simulink model "lqg_control"  (R2018a)
settings: Solver=ode45  StartTime=0.0  StopTime=10  RelTol=1e-3
settings Model: Creator=HARSH  LastModifiedBy=HARSH

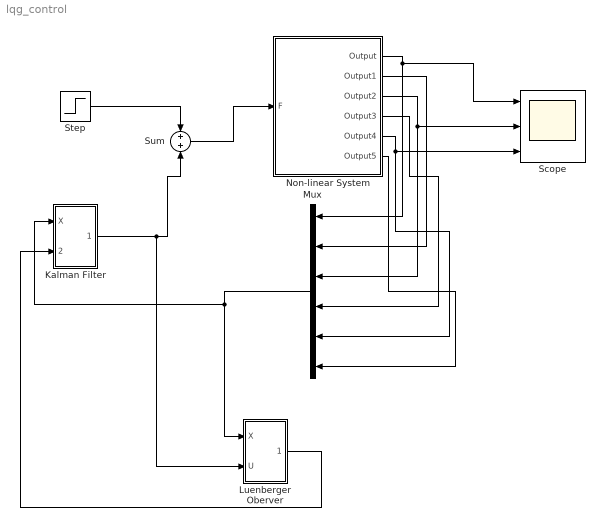
== system lqg_control ==
  "Kalman Filter " : Subsystem
  Luenberger Oberver : Subsystem
  Mux : Mux  Inputs=6
  Non-linear System : Subsystem
  Scope : Scope  NumInputPorts=3
  Step : Step  After=20  SampleTime=0
  Sum : Sum  Inputs=2
  wires:
  Non-linear System/1(Output) -> Scope/1, Mux/1
  Non-linear System/2(Output1) -> Mux/2
  Non-linear System/3(Output2) -> Scope/2, Mux/3
  Non-linear System/4(Output3) -> Mux/4
  Non-linear System/6(Output5) -> Mux/6
  Mux/1 -> "Kalman Filter "/1(X), Luenberger Oberver/1(X)
  Sum/1 -> Non-linear System/1(F)
  Step/1 -> Sum/1
  "Kalman Filter "/1(Out1) -> Luenberger Oberver/2(U), Sum/2
  Luenberger Oberver/1(X_hat) -> "Kalman Filter "/2(X_hat)
  Non-linear System/5(Output4) -> Scope/3, Mux/5

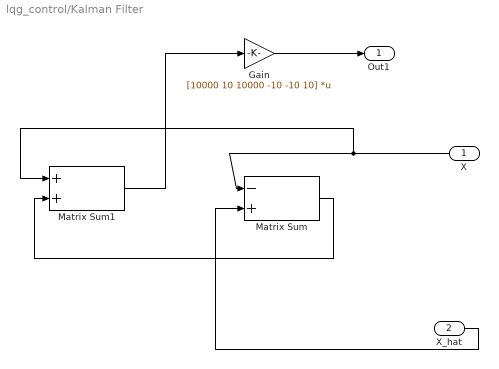
== system lqg_control/Kalman Filter  ==
  X : Inport
  X_hat : Inport  Port=2
  Gain : Gain  Gain=[10000 10 10000 -10 -10 10]  Multiplication=Matrix(K*u)
  Matrix Sum : Sum  Inputs=-+
  Matrix Sum1 : Sum  Inputs=2
  Out1 : Outport
  wires:
  X_hat/1 -> Matrix Sum/2
  Gain/1 -> Out1/1
  X/1 -> Matrix Sum1/1, Matrix Sum/1
  Matrix Sum/1 -> Matrix Sum1/2
  Matrix Sum1/1 -> Gain/1

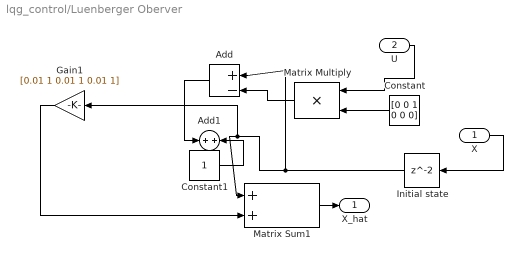
== system lqg_control/Luenberger Oberver ==
  X : Inport
  U : Inport  Port=2
  Add : Sum  Inputs=+|-
  Add1 : Sum
  Constant : Constant  Value=[0 0 1 0 0 0]  VectorParams1D=off
  Constant1 : Constant
  Gain1 : Gain  Gain=[0.01 1 0.01 1 0.01 1]
  Initial state : Delay  InitialCondition=1  SampleTime=0.001
  Matrix Sum1 : Sum  Inputs=2
  Matrix Multiply : Product  Inputs=**  OutMin=0  OutMax=0
  X_hat : Outport
  wires:
  Matrix Sum1/1 -> X_hat/1
  X/1 -> Initial state/1
  Constant/1 -> Matrix Multiply/2
  U/1 -> Matrix Multiply/1
  Initial state/1 -> Add/1, Gain1/1, Matrix Sum1/1
  Gain1/1 -> Matrix Sum1/2
  Matrix Multiply/1 -> Add/2
  Add/1 -> Add1/1
  Constant1/1 -> Add1/2

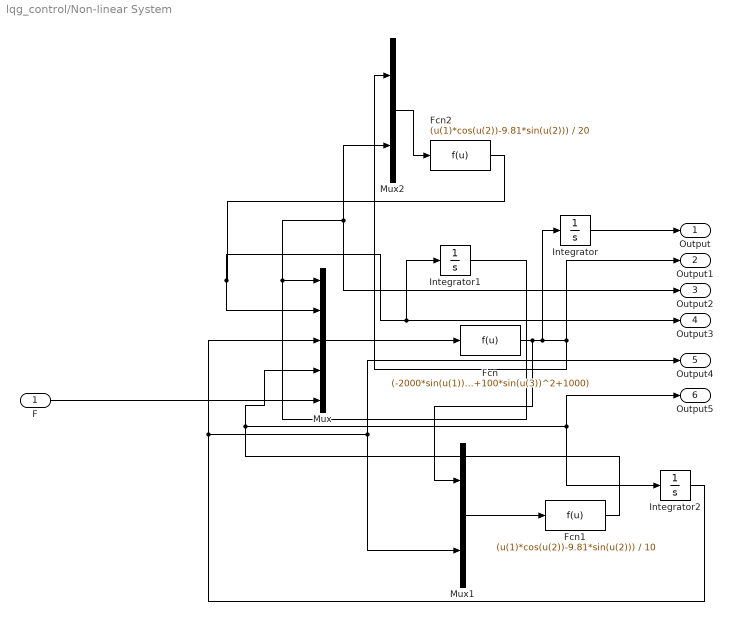
== system lqg_control/Non-linear System ==
  F : Inport
  Fcn : Fcn  Expr=(-2000*sin(u(1))*u(2)^2 + 1000*sin(u(3))*u(4)^2-u(5)+981*cos(u(1))*sin(u(1))+981*cos(u(3))*sin(u(3)))/(100*sin(u(1))^2+100*sin(u(3))^2+1000)
  Fcn1 : Fcn  Expr=(u(1)*cos(u(2))-9.81*sin(u(2))) / 10
  Fcn2 : Fcn  Expr=(u(1)*cos(u(2))-9.81*sin(u(2))) / 20
  Integrator : Integrator  InitialCondition=-2
  Integrator1 : Integrator  InitialCondition=-.5
  Integrator2 : Integrator  InitialCondition=-.5  ZeroCross=off
  Mux : Mux  Inputs=5
  Mux1 : Mux  Inputs=2
  Mux2 : Mux  Inputs=2
  Output : Outport
  Output1 : Outport  Port=2
  Output2 : Outport  Port=3
  Output3 : Outport  Port=4
  Output4 : Outport  Port=5
  Output5 : Outport  Port=6
  wires:
  Fcn/1 -> Mux1/1, Integrator/1, Output1/1, Mux2/1
  F/1 -> Mux/5
  Integrator/1 -> Output/1
  Integrator2/1 -> Mux/3, Output4/1, Mux1/2
  Mux1/1 -> Fcn1/1
  Integrator1/1 -> Output2/1, Mux2/2, Mux/1
  Fcn1/1 -> Mux/4, Output5/1, Integrator2/1
  Mux2/1 -> Fcn2/1
  Fcn2/1 -> Mux/2, Output3/1, Integrator1/1
  Mux/1 -> Fcn/1
